simulink model "Pratica8AnaliseSimulink"  (R2020a)
settings: Solver=VariableStepAuto  StartTime=0.0  StopTime=20  RelTol=1e-3
settings Model: Creator=xalin  LastModifiedBy=laris

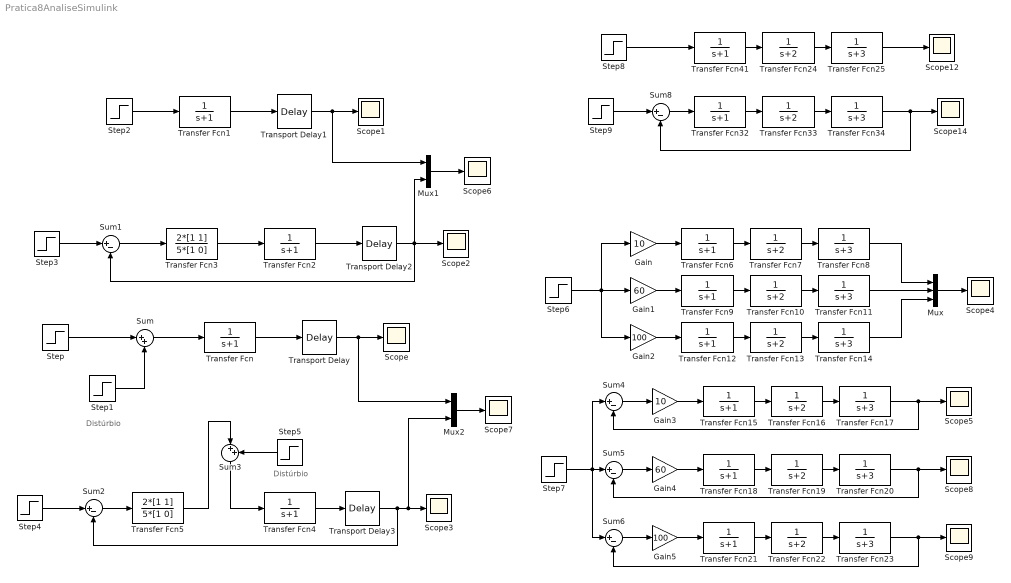
== system Pratica8AnaliseSimulink ==
  note: Distúrbio
  note: Distúrbio
  Gain : Gain  Gain=10
  Gain1 : Gain  Gain=60
  Gain2 : Gain  Gain=100
  Gain3 : Gain  Gain=10
  Gain4 : Gain  Gain=60
  Gain5 : Gain  Gain=100
  Mux : Mux  Inputs=3
  Mux1 : Mux  Inputs=2
  Mux2 : Mux  Inputs=2
  Scope{,1..9,12,14} (12 alike) : Scope
  Step{,2..4,6..9} (8 alike) : Step  SampleTime=0
  Step1 : Step  Time=10  After=0.3  SampleTime=0
  Step5 : Step  Time=10  After=0.3  SampleTime=0
  Sum : Sum  Inputs=|++
  Sum{1..2,4..6,8} (6 alike) : Sum  Inputs=|+-
  Sum3 : Sum  Inputs=|++
  Transfer Fcn{,1..2,4,6,9,12,15,18,21,32,41} (12 alike) : TransferFcn  Denominator=[1 1]
  Transfer Fcn{7,10,13,16,19,22,24,33} (8 alike) : TransferFcn  Denominator=[1 2]
  Transfer Fcn{8,11,14,17,20,23,25,34} (8 alike) : TransferFcn  Denominator=[1 3]
  Transfer Fcn3 : TransferFcn  Numerator=2*[1 1]  Denominator=5*[1 0]
  Transfer Fcn5 : TransferFcn  Numerator=2*[1 1]  Denominator=5*[1 0]
  Transport Delay{,1..3} (4 alike) : TransportDelay
  wires:
  Transport Delay/1 -> Mux2/1, Scope/1
  Transfer Fcn/1 -> Transport Delay/1
  Sum/1 -> Transfer Fcn/1
  Step1/1 -> Sum/2
  Step/1 -> Sum/1
  Transfer Fcn1/1 -> Transport Delay1/1
  Transport Delay1/1 -> Mux1/1, Scope1/1
  Step2/1 -> Transfer Fcn1/1
  Transfer Fcn2/1 -> Transport Delay2/1
  Transport Delay2/1 -> Mux1/2, Scope2/1, Sum1/2
  Transfer Fcn3/1 -> Transfer Fcn2/1
  Step3/1 -> Sum1/1
  Sum1/1 -> Transfer Fcn3/1
  Step4/1 -> Sum2/1
  Sum2/1 -> Transfer Fcn5/1
  Transfer Fcn4/1 -> Transport Delay3/1
  Transport Delay3/1 -> Sum2/2, Mux2/2, Scope3/1
  Sum3/1 -> Transfer Fcn4/1
  Step5/1 -> Sum3/2
  Transfer Fcn5/1 -> Sum3/1
  Sum4/1 -> Gain3/1
  Transfer Fcn6/1 -> Transfer Fcn7/1
  Transfer Fcn7/1 -> Transfer Fcn8/1
  Gain/1 -> Transfer Fcn6/1
  Transfer Fcn9/1 -> Transfer Fcn10/1
  Transfer Fcn10/1 -> Transfer Fcn11/1
  Transfer Fcn11/1 -> Mux/2
  Gain1/1 -> Transfer Fcn9/1
  Transfer Fcn12/1 -> Transfer Fcn13/1
  Transfer Fcn13/1 -> Transfer Fcn14/1
  Transfer Fcn14/1 -> Mux/3
  Gain2/1 -> Transfer Fcn12/1
  Step6/1 -> Gain1/1, Gain/1, Gain2/1
  Gain3/1 -> Transfer Fcn15/1
  Transfer Fcn15/1 -> Transfer Fcn16/1
  Transfer Fcn16/1 -> Transfer Fcn17/1
  Transfer Fcn17/1 -> Sum4/2, Scope5/1
  Gain4/1 -> Transfer Fcn18/1
  Sum5/1 -> Gain4/1
  Transfer Fcn19/1 -> Transfer Fcn20/1
  Transfer Fcn18/1 -> Transfer Fcn19/1
  Transfer Fcn20/1 -> Sum5/2, Scope8/1
  Gain5/1 -> Transfer Fcn21/1
  Sum6/1 -> Gain5/1
  Transfer Fcn22/1 -> Transfer Fcn23/1
  Transfer Fcn21/1 -> Transfer Fcn22/1
  Transfer Fcn23/1 -> Sum6/2, Scope9/1
  Step7/1 -> Sum6/1, Sum4/1, Sum5/1
  Step8/1 -> Transfer Fcn41/1
  Transfer Fcn41/1 -> Transfer Fcn24/1
  Transfer Fcn25/1 -> Scope12/1
  Step9/1 -> Sum8/1
  Transfer Fcn24/1 -> Transfer Fcn25/1
  Transfer Fcn32/1 -> Transfer Fcn33/1
  Transfer Fcn33/1 -> Transfer Fcn34/1
  Sum8/1 -> Transfer Fcn32/1
  Transfer Fcn34/1 -> Sum8/2, Scope14/1
  Mux/1 -> Scope4/1
  Transfer Fcn8/1 -> Mux/1
  Mux2/1 -> Scope7/1
  Mux1/1 -> Scope6/1
